simulink model "forward_converter"  (R2018a)
settings: Solver=VariableStepAuto  StartTime=0.0  StopTime=0.05  MaxStep=1e-6  RelTol=1e-3
libraries: powerlib x14, powerlib_meascontrol x3
settings Model: Creator=Ogün Altun  LastModifiedBy=Ogün Altun

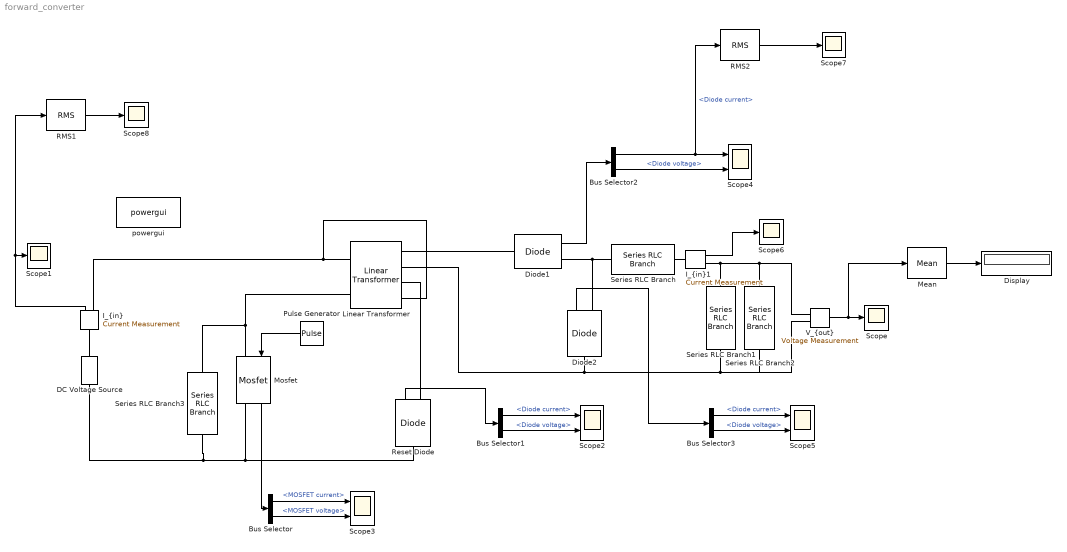
== system forward_converter ==
  Bus Selector : BusSelector  OutputSignals=MOSFET current,MOSFET voltage
  Bus Selector1 : BusSelector  OutputSignals=Diode current,Diode voltage
  Bus Selector2 : BusSelector  OutputSignals=Diode current,Diode voltage
  Bus Selector3 : BusSelector  OutputSignals=Diode current,Diode voltage
  DC Voltage Source : powerlib/Electrical Sources/DC Voltage Source  Amplitude=24  Measurements=None
  Diode1 : powerlib/Power Electronics/Diode  Ron=0.001  Lon=0  Vf=0.75  IC=0  UseSnubber=0  Rs=inf  Cs=0  Measurements=on
  Diode2 : powerlib/Power Electronics/Diode  Ron=0.001  Lon=0  Vf=0.75  IC=0  UseSnubber=0  Rs=inf  Cs=0  Measurements=on
  Display : Display
  "I_{in}" : powerlib/Measurements/Current Measurement  PhasorSimulation=off  OutputType=Complex  PSBequivalent=0
  "I_{in}1" : powerlib/Measurements/Current Measurement  PhasorSimulation=off  OutputType=Complex  PSBequivalent=0
  Linear Transformer : powerlib/Elements/Linear Transformer  UNITS=SI  NominalPower=[48 40000]  winding1=[48 0.0214 3e-5]  winding2=[48 0.0214 0]  ThreeWindings=on  winding3=[48 0.0642 0]  RmLm=[1e5 2e-3]  Measurements=None  DataType=on
  Mean : powerlib_meascontrol/Measurements/Mean  Freq=20000  Vinit=0  Ts=0
  Mosfet : powerlib/Power Electronics/Mosfet  Ron=0.18  Lon=0  Rd=0.0001  Vfd=1.5  IC=0  Rs=inf  Cs=inf  Measurements=on
  Pulse Generator : DiscretePulseGenerator  PulseType=Time based  Amplitude=5  Period=1/40000  PulseWidth=46
  RMS1 : powerlib_meascontrol/Measurements/RMS  TrueRMS=on  Freq=40000  RMSInit=120  Ts=0
  RMS2 : powerlib_meascontrol/Measurements/RMS  TrueRMS=on  Freq=40000  RMSInit=120  Ts=0
  Reset Diode : powerlib/Power Electronics/Diode  Ron=0.001  Lon=0  Vf=0.87  IC=0  UseSnubber=0  Rs=inf  Cs=0  Measurements=on
  Scope{,1,6..8} (5 alike) : Scope
  Scope{2..5} (4 alike) : Scope  NumInputPorts=2
  Series RLC Branch : powerlib/Elements/Series RLC Branch  LConnTagsString=__new0  RConnTagsString=__new0  BranchType=RL  Resistance=0.03683  Inductance=500e-6  SetiL0=off  InitialCurrent=0  Capacitance=1e-6  Setx0=off  InitialVoltage=0  Measurements=None
  Series RLC Branch1 : powerlib/Elements/Series RLC Branch  LConnTagsString=__new0  RConnTagsString=__new0  BranchType=C  Resistance=1.5e-3  Inductance=1e-3  SetiL0=off  InitialCurrent=0  Capacitance=220e-6  Setx0=off  InitialVoltage=0  Measurements=None
  Series RLC Branch2 : powerlib/Elements/Series RLC Branch  LConnTagsString=__new0  RConnTagsString=__new0  BranchType=R  Resistance=2.0833  Inductance=1e-3  SetiL0=off  InitialCurrent=0  Capacitance=1e-6  Setx0=off  InitialVoltage=0  Measurements=None
  Series RLC Branch3 : powerlib/Elements/Series RLC Branch  LConnTagsString=__new0  RConnTagsString=__new0  BranchType=RC  Resistance=10  Inductance=500e-6  SetiL0=off  InitialCurrent=0  Capacitance=1e-5  Setx0=off  InitialVoltage=0  Measurements=None
  "V_{out}" : powerlib/Measurements/Voltage Measurement  PhasorSimulation=off  OutputType=Complex  PSBequivalent=0
  powergui : powerlib/powergui  Priority=1  SimulationMode=Continuous  SampleTime=50e-6  frequency=60  Iterations=50  frequencyindice=0  Pbase=100e6  ErrMax=1e-4  UnitsV=kV  UnitsW=MW  buscounter=0  FunctionMessages=off  echomessages=off  EnableUseOfTLC=off  CurrentSourceSwitches=off  DisableSnubberDevices=off  DisableRonSwitches=off  DisableVfSwitches=off  DisplayEquations=off  SolverType=Tustin/Backward Euler (TBE)  Interpol=off  ExternalGateDelay=off  methode=off  Ts=100  x0status=blocks  SPID=on  SwTol=0  HookPort=off  RestoreLinks=warning  ResistiveCurrentMeasurement=off  Frange=[0:2:500]  Ylog=off  Xlog=on  ShowGrid=off  save=off  variable=ZData  structure=0  ZoomFFT=off  StartTime=0.0  cycles=1  DisplayStyle=1  fundamental=60  FreqAxis=off  MaxFrequency=1000  frequencyindicesteady=1  RmsSteady=1  display=off
  wires:
  "V_{out}"/1 -> Mean/1, Scope/1
  Pulse Generator/1 -> Mosfet/1
  Mosfet/1 -> Bus Selector/1
  Bus Selector/1 -> Scope3/1  "<MOSFET current>"
  Bus Selector/2 -> Scope3/2  "<MOSFET voltage>"
  Bus Selector1/1 -> Scope2/1  "<Diode current>"
  Bus Selector1/2 -> Scope2/2  "<Diode voltage>"
  Reset Diode/1 -> Bus Selector1/1
  Bus Selector2/2 -> Scope4/2  "<Diode voltage>"
  Diode1/1 -> Bus Selector2/1
  Bus Selector2/1 -> RMS2/1, Scope4/1  "<Diode current>"
  Bus Selector3/2 -> Scope5/2  "<Diode voltage>"
  Diode2/1 -> Bus Selector3/1
  Bus Selector3/1 -> Scope5/1  "<Diode current>"
  Mean/1 -> Display/1
  "I_{in}1"/1 -> Scope6/1
  RMS2/1 -> Scope7/1
  RMS1/1 -> Scope8/1
  "I_{in}"/1 -> RMS1/1, Scope1/1
  connections:
  Series RLC Branch2/LConn1 -- "V_{out}"/LConn1 -- "I_{in}1"/RConn1 -- Series RLC Branch1/LConn1
  DC Voltage Source/LConn1 -- Series RLC Branch3/RConn1 -- Mosfet/RConn1 -- Reset Diode/LConn1
  "I_{in}"/RConn1 -- Linear Transformer/RConn4 -- Linear Transformer/LConn1
  Linear Transformer/LConn2 -- Series RLC Branch3/LConn1 -- Mosfet/LConn1
  Diode2/RConn1 -- Series RLC Branch/LConn1 -- Diode1/RConn1
  Series RLC Branch2/RConn1 -- "V_{out}"/LConn2 -- Linear Transformer/RConn2 -- Diode2/LConn1 -- Series RLC Branch1/RConn1
  "I_{in}"/LConn1 -- DC Voltage Source/RConn1
  Linear Transformer/RConn1 -- Diode1/LConn1
  Linear Transformer/RConn3 -- Reset Diode/RConn1
  "I_{in}1"/LConn1 -- Series RLC Branch/RConn1
